simulink model "SimscapeSystemLevel_e8_IPMSM_HWJandVent_ROM"  (R2021b)
settings: Solver=VariableStepAuto  StartTime=0.0  StopTime=300  FixedStep=1  RelTol=1e-3  AbsTol=1e-3
model workspace (MAT data in the model file):
  AdjacencyMat = [0 0 0 0 0 0 0 0 0 0 0 0 ... (15129 elements, 123x123)]
  CapMat = [1e+20; 2196.70091586; 387.653102799; 193.8265514; 1962.34710525; 387.653102799; 193.8265514; 1962.34710525; 1266.59353814; 268.053957132; 416.539515956; 175.715078; 577.243160678; 310.101557898; 23.9530731873; 15.4990473565; 47.9061463746; 30.998094713; 85.98384; 1.11955442905; 1.11955442905; 1.11955442905; 1.11955442905; 1.11955442905; 1.11955442905; 0.373184809682; 0.373184809682; 450.202206395; 54.9511679003; 54.9511679003; 247.389926005; 247.389926005; 75.306462; 75.306462; 1.11955442905; 1.11955442905; 1e+20; 1e+20; 0; 0; 0; 0; 429.469897824; 0; 0; 0; 0; 429.469897824; 0; 0; 0; 0; 0; 0; 424.408023296; 268.053957132; 0; 0; 0; 0; 0; 322.102423368; 0; 0; 0; 0; 0; 322.102423368; 0; 0; 0; 0; 0; 318.306017472; 268.053957132; 2196.70091586; 1266.59353814; 268.053957132; 416.539515956; 175.715078; 577.243160678; 310.101557898; 85.98384; 0.373184809682; 0.373184809682; 450.202206395; 0; 0; 0; 0; 0; 424.408023296; 268.053957132; 0; 0; 0; 0; 318.306017472; 268.053957132; 2196.70091586; 1266.59353814; 268.053957132; 416.539515956; 175.715078; 577.243160678; 310.101557898; 85.98384; 0.373184809682; 0.373184809682; 450.202206395; 0; 0; 0; 0; 0; 424.408023296; 268.053957132; 0; 0; 0; 0; 318.306017472; 268.053957132]
  CoolantArrayIdxs = [20; 21; 22; 23; 24; 25; 26; 27; 35; 36; 37; 84; 85; 108; 109; 19; 38; 83; 107]
  Friction_Loss_Mat = [0 0 0 0 0 0 0 0 0 0 0 0 ... (2340 elements, 39x60)]
  InletCoolIdxs = [37; 38]
  Iron_Loss_Rotor_Back_Iron_Mat = [0.0117705351991 0.0198175800092 0.0246057415963 0.0256631766661 0.0240576767285 0.0207771722396 0.0168311502834 0.0133395315761 0.0115512535049 0.0120779527774 0.0143067244388 0.0171516443454 ... (2340 elements, 39x60)]
  Iron_Loss_Rotor_Pole_Mat = [1.45649756865 1.4525095653 1.42942652973 1.39109338754 1.34251579982 1.287439524 1.22885659237 1.16930852698 1.11098912611 1.05484046499 0.999976047808 0.944563732162 ... (2340 elements, 39x60)]
  Iron_Loss_Rotor_Tooth_Mat = [0 0 0 0 0 0 0 0 0 0 0 0 ... (2340 elements, 39x60)]
  Iron_Loss_Stator_Back_Iron_Mat = [38.5419456951 37.774471759 36.7837540443 35.6885758764 34.5272571596 33.3324529178 32.136302555 30.9744032473 29.8863152048 28.8790573391 27.8876077961 26.8074662049 ... (2340 elements, 39x60)]
  Iron_Loss_Stator_Tooth_Mat = [42.0610884508 41.0604961882 40.1804594162 39.4285940164 38.704339026 37.9602455604 37.1844153901 36.3902226975 35.6050856075 34.8287218867 34.0007237809 33.0439458619 ... (2340 elements, 39x60)]
  LossDistrForEachType = [0 0 0 0 0 0 0 0 0 0 0 0 ... (1968 elements, 16x123)]
  Magnet_Loss_Mat = [0.0995193918038 0.0928899922278 0.0868628846748 0.0818830115456 0.0774722500184 0.0732395922727 0.0687988836096 0.0636930921801 0.0573503948699 0.0496000064543 0.0410757743485 0.0326817704515 ... (2340 elements, 39x60)]
  OutletCoolIdxs = [20; 107]
  ResMat = [0 2.49009256841 6.64572241429 1000000000 1.39790968864 6.64402802995 1000000000 1.39156082742 1000000000 1000000000 1000000000 1000000000 ... (15129 elements, 123x123)]
  RotorCopperTempCoefResistivity = 0.00393
  Rotor_Cage_Loss_Mat = [0 0 0 0 0 0 0 0 0 0 0 0 ... (2340 elements, 39x60)]
  ShaftTorqueVec = [-287.262157301 -272.268610731 -257.275064161 -242.281517591 -227.287971021 -212.294424451 -197.300877881 -182.307331311 -167.31378474 -152.32023817 -137.3266916 -122.33314503 -107.33959846 -92.34605189 -77.35250532 -62.3589587499 -47.3654121798 -32.3718656097 -17.3783190396 -2.38477246955 12.6087741005 27.6023206706 42.5958672407 57.5894138108 72.5829603809 87.576506951 102.570053521 117.563600091 132.557146661 147.550693231 162.544239801 177.537786371 192.531332942 207.524879512 222.518426082 237.511972652 252.505519222 267.499065792 282.492612362]
  SpeedVec = [500 661.016949153 822.033898305 983.050847458 1144.06779661 1305.08474576 1466.10169492 1627.11864407 1788.13559322 1949.15254237 2110.16949153 2271.18644068 2432.20338983 2593.22033898 2754.23728814 2915.25423729 3076.27118644 3237.28813559 3398.30508475 3559.3220339 3720.33898305 3881.3559322 4042.37288136 4203.38983051 4364.40677966 4525.42372881 4686.44067797 4847.45762712 5008.47457627 5169.49152542 5330.50847458 5491.52542373 5652.54237288 5813.55932203 5974.57627119 6135.59322034 6296.61016949 6457.62711864 6618.6440678 6779.66101695 6940.6779661 7101.69491525 7262.71186441 7423.72881356 7584.74576271 7745.76271186 7906.77966102 8067.79661017 8228.81355932 8389.83050847 8550.84745763 8711.86440678 8872.88135593 9033.89830508 9194.91525424 9355.93220339 9516.94915254 9677.96610169 9838.98305085 10000]
  StateSpaceND : object (value not decoded)
  StatorCopperTempCoefResistivity = 0.00393
  Stator_Copper_Loss_Mat = [3925.33912093 3510.19452231 3089.33767218 2711.80000483 2370.99356953 2062.06508217 1781.35176729 1526.02799256 1293.87708125 1083.15658499 892.54525431 720.809889245 ... (2340 elements, 39x60)]
  Stray_Load_Loss_Mat = [0 0 0 0 0 0 0 0 0 0 0 0 ... (2340 elements, 39x60)]
  Stray_Loss_Stator_Iron_Proportion = 0.95
  Tgiven = 20
  TnodesInit = [25; 25; 25; 25; 25; 25; 25; 25; 25; 25; 25; 25; 25; 25; 25; 25; 25; 25; 25; 25; 25; 25; 25; 25; 25; 25; 25; 25; 25; 25; 25; 25; 25; 25; 25; 25; 25; 25; 25; 25; 25; 25; 25; 25; 25; 25; 25; 25; 25; 25; 25; 25; 25; 25; 25; 25; 25; 25; 25; 25; 25; 25; 25; 25; 25; 25; 25; 25; 25; 25; 25; 25; 25; 25; 25; 25; 25; 25; 25; 25; 25; 25; 25; 25; 25; 25; 25; 25; 25; 25; 25; 25; 25; 25; 25; 25; 25; 25; 25; 25; 25; 25; 25; 25; 25; 25; 25; 25; 25; 25; 25; 25; 25; 25; 25; 25; 25; 25; 25; 25; 25; 25; 25]
  TrefRotor = 20
  TrefStator = 20
  Windage_Loss_Mat = [0 0 0 0 0 0 0 0 0 0 0 0 ... (2340 elements, 39x60)]
libraries: fl_lib x33, nesl_utility x13, mcadROM_lib x4, simulink_extras x2, autolibshared x1, slpidlib x1, SimscapeFluids_lib x1
(part 1 of 2)
settings Model: Creator=agonzale  LastModifiedBy=agonzale
settings SolverCC: AutoScaleAbsTol=off  MaxConsecutiveZCs=100  MaxConsecutiveMinStep=10
settings SimscapeCC: SimscapeLogType=all  SimscapeLogDecimation=10  SimscapeLogLimitData=off

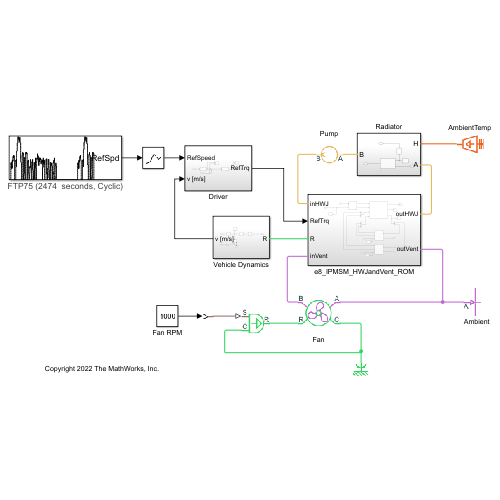
[thumbnail: Simulink's stored preview of the top-level diagram]
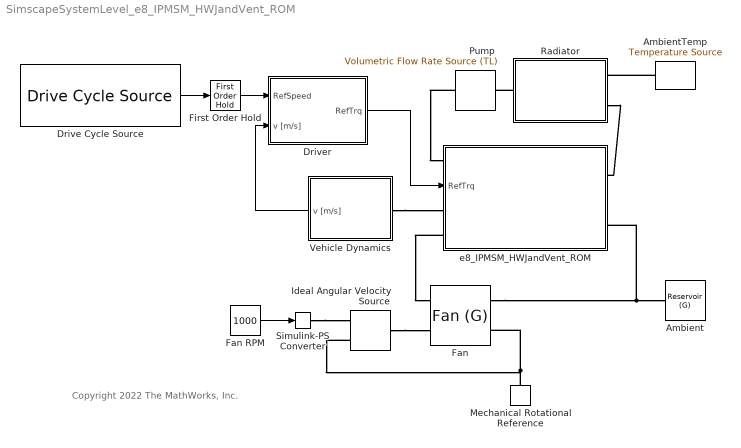
== system SimscapeSystemLevel_e8_IPMSM_HWJandVent_ROM ==
  note: Copyright 2022 The MathWorks, Inc.
  Ambient : fl_lib/Gas/Elements/Reservoir (G)  pressure_spec=foundation.enum.pressure_spec.atmospheric  reservoir_pressure=0.101325 MPa  reservoir_temperature=TnodesInit(1) degC  area_A=0.01 m^2
      settings: SourceProductBaseCode=SS
  AmbientTemp : fl_lib/Thermal/Thermal Sources/Temperature Source  temperature=TnodesInit(1) degC
  Drive Cycle Source : autolibshared/Drive Cycle Source  cycleVar=FTP75  fileVar=cycleFTP75.mat  tfinal="2474  seconds, Cyclic"  cycleRepeat=on  outAccPort=off  outGearPort=off  gearList=No gear data  t_wot1=5  xdot_woto=0  xdot_wot1=30  t_wot2=20  xdot_wot2=0  t_wotend=30  srcUnit=m/s  outUnit=m/s  srcAccUnit=m/s/s  outAccUnit=m/s^2  dt=5  aMode=2  faultOption=off  velBnd=2  velBndUnit=mph  inUnit=m/s  timeBnd=1  failOption=off  stopSim=off  maxFaultCnt=10  maxFaultTime=2  maxTotFaultTime=15  traceOption=off  dtTrace=1  traceWindow=10  lastDCname=FTP75  lastOutUnit=mph  lastDT=5  lastTB=1  lastSB=2  forceCalcBound=off
      settings: SourceProductBaseCode=PW,DR,MT,UV,VE
  Driver : Subsystem
  Fan : SimscapeFluids_lib/Gas/Turbomachinery/Fan (G)  fan_parameterization=fluids.gas.turbomachinery.enum.FanParameterization.Nominal  mechanical_power_spec=fluids.gas.turbomachinery.enum.FanMechanicalPowerSpec.Power  flow_rate_nominal=5 lpm  pressure_nominal=600 Pa  eta_nominal=0.40  power_nominal=10 W  pressure_max=1000 Pa  flow_rate_max=10 lpm  omega_ref_nominal=1000 rpm  flow_rate_1D_TLU=[.0278, .0556, .0833, .111, .139, .167] m^3/s  pressure_1D_TLU=[6410, 6375, 6018, 5366, 4501, 3609] Pa  eta_1D_TLU=[.257, .394, .453, .47, .459, .415]  power_1D_TLU=[693, 900, 1107, 1267, 1363, 1452] W  omega_ref_1D=3000 rpm  rho_ref_1D=1.2 kg/m^3  omega_dp_TLU=[2400; 3000; 3600] rpm  flow_rate_dp_TLU=[.0278, .0556, .0833, .111, .139, .167] m^3/s  pressure_dp_TLU=[4111, 4010, 3551, 2881, 2167, 1453; 6410, 6375, 6018, 5366, 4501, 3609; 9217, 9285, 9022, 8428, 7552, 6482] Pa  eta_dp_TLU=[.3, .434, .468, .459, .4, .3; .257, .394, .453, .47, .459, .415; .225, .359, .434, .461, .47, .459]  power_dp_TLU=[381, 514, 632, 697, 753, 809; 693, 900, 1107, 1267, 1363, 1452; 1139, 1438, 1732, 2029, 2233, 2358] W  rho_ref_dp=1.2 kg/m^3  omega_q_TLU=[2990; 3450; 3867] rpm  pressure_q_TLU=[31, 62, 93, 124] Pa  flow_rate_q_TLU=[.802, .759, .703, .611; .936, .902, .862, .81; 1.056, 1.027, .994, .956] m^3/s  eta_q_TLU=[.088, .162, .22, .261; .068, .128, .18, .222; .055, .105, .148, .188]  power_q_TLU=[283, 290, 297, 290; 427, 437, 445, 452; 595, 606, 625, 631] W  rho_ref_q=1.2 kg/m^3  diameter_ratio=1  mech_orientation=fluids.gas.turbomachinery.enum.FanMechanicalOrientation.Positive  area_A=0.01 m^2  area_B=0.01 m^2
      settings: SourceProductBaseCode=SH  InternalSimscapePortConfiguration="{\"Bottom\":[],\"Left\":[{\"id\":\"A\",\"label\":\"A\",\"type\":\"foundation.gas.gas\"},{\"id\":\"C\",\"label\":\"C\",\"type\":\"foundation.mechanical.rotational.rotational\"}],\"Right\":[{\"id\":\"B\",\"label\":\"B\",\"type\":\"foundation.gas.gas\"},{\"id\":\"R\",\"label\":\"R\",\"type\":\"foundation.mechanical.rotational.rotational\"}],\"Top\":[]}"
  Fan RPM : Constant  Value=1000
  First Order Hold : FirstOrderHold  ErrorTolerance=inf
  Ideal Angular Velocity Source : fl_lib/Mechanical/Mechanical Sources/Ideal Angular Velocity Source
  Mechanical Rotational Reference : fl_lib/Mechanical/Rotational Elements/Mechanical Rotational Reference
  Pump : fl_lib/Thermal Liquid/Sources/Volumetric Flow Rate Source (TL)  commanded_volumetric_flow=5 lpm  area=0.01 m^2
      settings: SourceProductBaseCode=SS  InternalSimscapePortConfiguration="{\"Bottom\":[],\"Left\":[{\"id\":\"A\",\"label\":\"A\",\"type\":\"foundation.thermal_liquid.thermal_liquid\"}],\"Right\":[{\"id\":\"B\",\"label\":\"B\",\"type\":\"foundation.thermal_liquid.thermal_liquid\"}],\"Top\":[]}"
  Radiator : Subsystem
  Simulink-PS Converter : nesl_utility/Simulink-PS Converter  PhysicalDomain=network_engine_domain  SubClassName=ps_input  LeftPortType=input  RightPortType=output  PseudoPeriodic=off  Frequencies=[]  NoiseDistribution=none  NoiseParameters=[]  Unit=rpm  AffineConversion=off  FilteringAndDerivatives=provide  SimscapeFilterOrder=1  InputFilterTimeConstant=0.001  UdotUserProvided=0
      settings: SourceProductBaseCode=PW,SS
  Vehicle Dynamics : Subsystem
      settings: PortSchema="{\"entries\":[{\"content\":{\"sides\":[{\"content\":{\"connectorIds\":[\"Out1\"]},\"type\":\"ConnectorPlacement.EquallySpacedRectSide\",\"uuid\":\"47062009-5743-4348-bd08-1dc005009362\"},{\"content\":{\"connectorIds\":[\"RConn1\"],\"side\":\"RIGHT\"},\"type\":\"ConnectorPlacement.EquallySpacedRectSide\",\"uuid\":\"e584846c-37d6-4d4a-a7bb-9d030c09d6b0\"},{\"content\":{\"connectorIds\":[],\"side\":\"TOP\"},\"type\":\"ConnectorPlacement.EquallySpacedRectSide\",\"uuid\":\"782dfd52-d1c7-40c0-b4f0-84ad0cd39623\"}]},\"type\":\"ConnectorPlacement.EquallySpacedConnector\",\"uuid\":\"2cc4fcb1-3940-4b3e-9118-d9ba66018413\"}],\"packageUris\":[\"http://schema.mathworks.com/mf0/Connector/R2020b\"],\"version\":\"1.0\"}"
  e8_IPMSM_HWJandVent_ROM : Subsystem
      settings: PortSchema="{\"entries\":[{\"content\":{\"sides\":[{\"content\":{\"connectorIds\":[\"LConn1\",\"In1\",\"LConn2\",\"LConn3\"]},\"type\":\"ConnectorPlacement.EquallySpacedRectSide\",\"uuid\":\"cefdaf80-ea7f-4720-b8ad-afd2aa86ff21\"},{\"content\":{\"connectorIds\":[\"RConn1\",\"RConn2\"],\"side\":\"RIGHT\"},\"type\":\"ConnectorPlacement.EquallySpacedRectSide\",\"uuid\":\"da03b82d-542b-4366-9583-37ca822c776b\"},{\"content\":{\"connectorIds\":[],\"side\":\"TOP\"},\"type\":\"ConnectorPlacement.EquallySpacedRectSide\",\"uuid\":\"feefb370-ce15-43ce-98e7-0cb1a3564374\"}]},\"type\":\"ConnectorPlacement.EquallySpacedConnector\",\"uuid\":\"f1cb3941-846e-48b7-8150-130b06fe1c99\"}],\"packageUris\":[\"http://schema.mathworks.com/mf0/Connector/R2020b\"],\"version\":\"1.0\"}"
  wires:
  Fan RPM/1 -> Simulink-PS Converter/1
  Drive Cycle Source/1 -> First Order Hold/1
  Driver/1(RefTrq) -> e8_IPMSM_HWJandVent_ROM/1(RefTrq)
  Vehicle Dynamics/1(v [m/s]) -> Driver/2(v [m/s])
  First Order Hold/1 -> Driver/1(RefSpeed)
  connections:
  Ideal Angular Velocity Source/LConn1 -- Fan/RConn2
  Mechanical Rotational Reference/LConn1 -- Fan/LConn2 -- Ideal Angular Velocity Source/RConn2
  Simulink-PS Converter/RConn1 -- Ideal Angular Velocity Source/RConn1
  AmbientTemp/LConn1 -- Radiator/LConn1
  Radiator/RConn1 -- Pump/LConn1
  e8_IPMSM_HWJandVent_ROM/LConn3 -- Fan/RConn1
  Pump/RConn1 -- e8_IPMSM_HWJandVent_ROM/LConn1
  Fan/LConn1 -- e8_IPMSM_HWJandVent_ROM/RConn2 -- Ambient/LConn1
  Radiator/LConn2 -- e8_IPMSM_HWJandVent_ROM/RConn1
  Vehicle Dynamics/RConn1 -- e8_IPMSM_HWJandVent_ROM/LConn2
